simulink model "msd_04_Simulink_4"  (R2026a)
settings: Solver=VariableStepAuto  MaxStep=0.01  AbsTol=1e-3
InitFcn:
  | m = 3.600;  % kg
  | k = 400;    % N/m
  | b = 10;     % Ns/m
Description:
  | Copyright 2017-2026 The MathWorks, Inc.
settings Model: Creator=smiller  LastModifiedBy=smiller
settings ConfigComp: CovMetricSettings=dswe
settings SimscapeCC: SimscapeNormalizeSystem=off  SimscapeNominalValues="[{\"value\":\"1\",\"unit\":\"A\"},{\"value\":\"1\",\"unit\":\"bar\"},{\"value\":\"1\",\"unit\":\"cm^2\"},{\"value\":\"1\",\"unit\":\"cm^3/s\"},{\"value\":\"1\",\"unit\":\"kJ/kg\"},{\"value\":\"1\",\"unit\":\"kW\"},{\"value\":\"1\",\"unit\":\"l\"},{\"value\":\"1\",\"unit\":\"N\"},{\"value\":\"1\",\"unit\":\"N*m\"},{\"value\":\"1\",\"unit\":\"V\"}]"

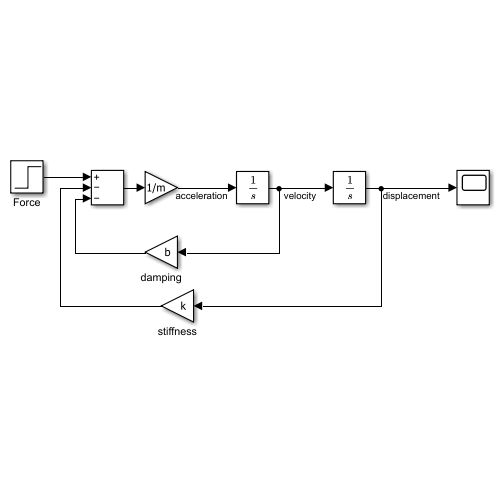
[thumbnail: Simulink's stored preview of the top-level diagram]
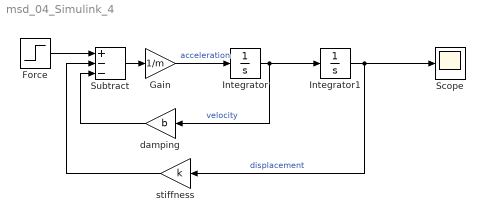
== system msd_04_Simulink_4 ==
  Force : Step  FinalValue=10  SampleTime=0
  Gain : Gain  Gain=1/m
  Integrator : Integrator
  Integrator1 : Integrator
  Scope : Scope
      settings: ActiveDisplayYMinimum=-0.00518  ActiveDisplayYMaximum=0.04665
  Subtract : Sum  Inputs=+--
  damping : Gain  Gain=b
  stiffness : Gain  Gain=k
  wires:
  Subtract/1 -> Gain/1
  Gain/1 -> Integrator/1  "acceleration"
  Integrator/1 -> damping/1, Integrator1/1  "velocity"
  Integrator1/1 -> stiffness/1, Scope/1  "displacement"
  damping/1 -> Subtract/3
  stiffness/1 -> Subtract/2
  Force/1 -> Subtract/1
